simulink model "c12_adaptiveDelay"  (R2022b)
settings: Solver=VariableStepAuto  StartTime=0.0  StopTime=20  RelTol=1e-3
values from neighbouring files (symbols this model uses):
  a0 = 1/5    (= 0.2)    [c12_delayAdaptive.m]
  gamma = out.ScopeData{2}.Values.Data    [c12_delayAdaptive.m]
  tau = 1    [c12_delayAdaptive.m]
  x0 = 5    [c12_delayAdaptive.m]    (also in c14_bipartite_MWconsensus_animation.m = [x0;r/norm(r)]; c15_closed_model.m = 5*rand(15,1); c15_open_model.m = 5*rand(15,1))
settings Model: Creator=trinh  LastModifiedBy=trinh

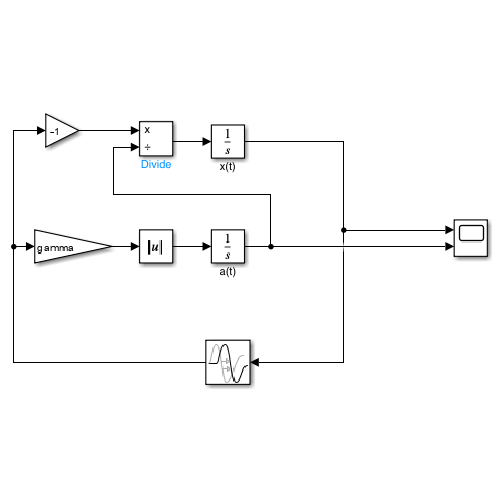
[thumbnail: Simulink's stored preview of the top-level diagram]
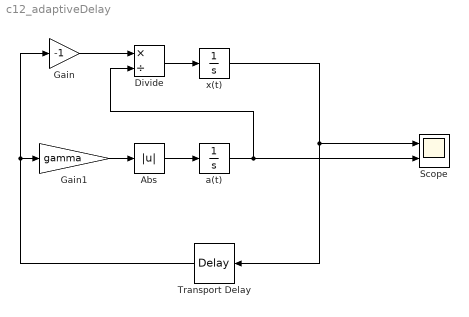
== system c12_adaptiveDelay ==
  Abs : Abs  SaturateOnIntegerOverflow=off
  Divide : Product  Inputs=*/
  Gain : Gain  Gain=-1
  Gain1 : Gain  Gain=gamma
  Scope : Scope  NumInputPorts=2
  Transport Delay : TransportDelay  DelayTime=tau
  a(t) : Integrator  InitialCondition=a0
  x(t) : Integrator  InitialCondition=x0
  wires:
  Divide/1 -> x(t)/1
  x(t)/1 -> Scope/1, Transport Delay/1
  Transport Delay/1 -> Gain1/1, Gain/1
  Abs/1 -> a(t)/1
  a(t)/1 -> Scope/2, Divide/2
  Gain/1 -> Divide/1
  Gain1/1 -> Abs/1
